simulink model "exercise1"  (R2021b)
settings: Solver=VariableStepAuto  StartTime=0.0  StopTime=t_f  RelTol=1e-3
values from neighbouring files (symbols this model uses):
  G_d = [1 0.12 1]    [Simulink_exercise_01.m]
  G_n = [0 1 1]    [Simulink_exercise_01.m]
  T_s = 0.01    [Simulink_exercise_01.m]
settings Model: Creator=Vincent Ryan  LastModifiedBy=Vincent Ryan

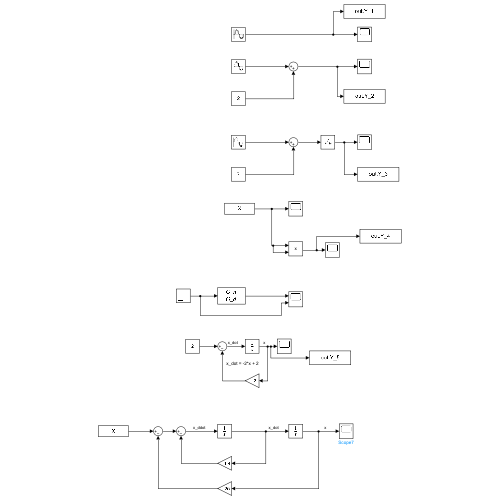
[thumbnail: Simulink's stored preview of the top-level diagram]
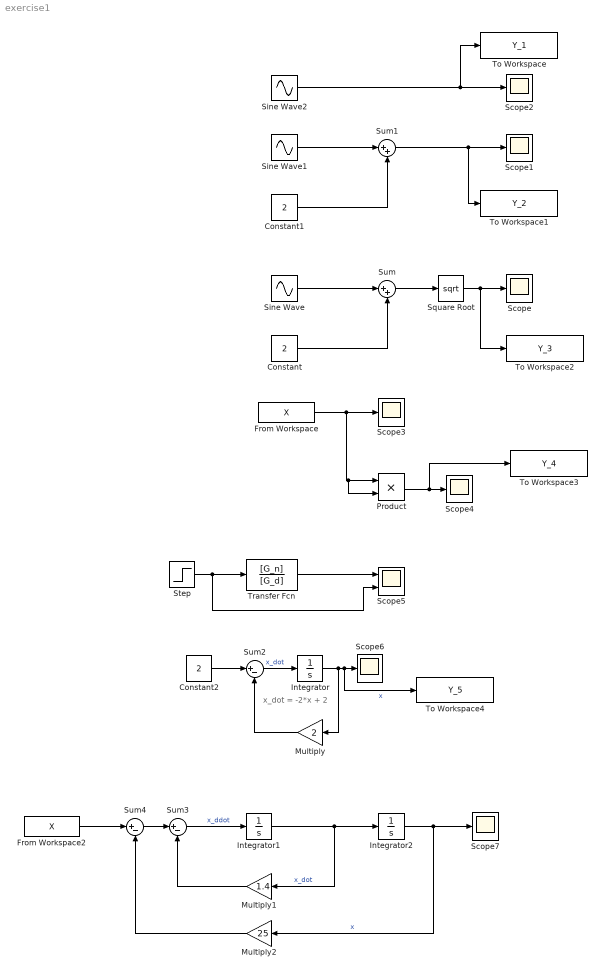
== system exercise1 ==
  note: x_dot = -2*x + 2
  Constant : Constant  Value=2
  Constant1 : Constant  Value=2
  Constant2 : Constant  Value=2
  From Workspace : FromWorkspace  VariableName=X  SampleTime=T_s
  From Workspace2 : FromWorkspace  VariableName=X  SampleTime=T_s
  Integrator : Integrator
  Integrator1 : Integrator
  Integrator2 : Integrator
  Multiply : Gain  Gain=2
  Multiply1 : Gain  Gain=1.4
  Multiply2 : Gain  Gain=25
  Product : Product
  Scope{,1..4,6..7} (7 alike) : Scope
  Scope5 : Scope  NumInputPorts=2
  Sine Wave : Sin  Amplitude=2  Frequency=2*pi  SampleTime=T_s
  Sine Wave1 : Sin  Amplitude=2  Frequency=2*pi  SampleTime=T_s
  Sine Wave2 : Sin  Amplitude=2  Frequency=2*pi  SampleTime=T_s
  Square Root : Sqrt  SaturateOnIntegerOverflow=on
  Step : Step  SampleTime=0
  Sum : Sum  Inputs=|++
  Sum1 : Sum  Inputs=|++
  Sum2 : Sum  Inputs=|+-
  Sum3 : Sum  Inputs=|+-
  Sum4 : Sum  Inputs=|+-
  To Workspace : ToWorkspace  VariableName=Y_1  SampleTime=T_s
  To Workspace1 : ToWorkspace  VariableName=Y_2  SampleTime=T_s
  To Workspace2 : ToWorkspace  VariableName=Y_3  SampleTime=T_s
  To Workspace3 : ToWorkspace  VariableName=Y_4  SampleTime=T_s
  To Workspace4 : ToWorkspace  VariableName=Y_5  SampleTime=T_s
  Transfer Fcn : TransferFcn  Numerator=[G_n]  Denominator=[G_d]
  wires:
  Sine Wave/1 -> Sum/1
  Constant/1 -> Sum/2
  Sum/1 -> Square Root/1
  Square Root/1 -> To Workspace2/1, Scope/1
  Sine Wave1/1 -> Sum1/1
  Constant1/1 -> Sum1/2
  Sum1/1 -> To Workspace1/1, Scope1/1
  Sine Wave2/1 -> To Workspace/1, Scope2/1
  From Workspace/1 -> Product/2, Product/1, Scope3/1
  Product/1 -> To Workspace3/1, Scope4/1
  Step/1 -> Scope5/2, Transfer Fcn/1
  Transfer Fcn/1 -> Scope5/1
  Constant2/1 -> Sum2/1
  Sum2/1 -> Integrator/1  "x_dot"
  Integrator/1 -> Multiply/1, To Workspace4/1, Scope6/1  "x"
  Multiply/1 -> Sum2/2
  Integrator1/1 -> Multiply1/1, Integrator2/1  "x_dot"
  Integrator2/1 -> Multiply2/1, Scope7/1  "x"
  Sum3/1 -> Integrator1/1  "x_ddot"
  Multiply1/1 -> Sum3/2
  Multiply2/1 -> Sum4/2
  Sum4/1 -> Sum3/1
  From Workspace2/1 -> Sum4/1
